simulink model "Task08_Model_Smith"  (R2026a)
settings: Solver=VariableStepAuto
settings Model: Creator=Tommy  LastModifiedBy=Tommy

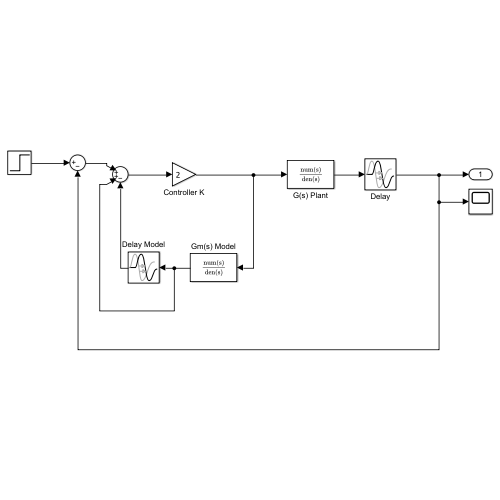
[thumbnail: Simulink's stored preview of the top-level diagram]
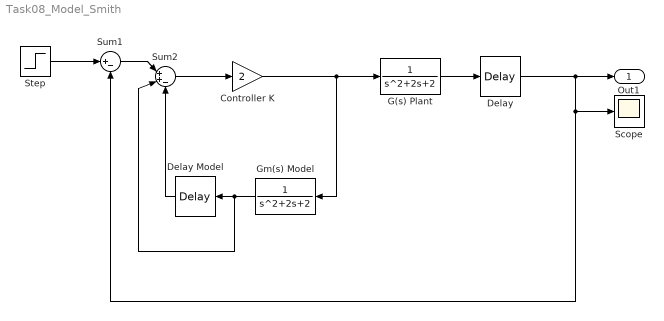
== system Task08_Model_Smith ==
  Controller K : Gain  Gain=2
  Delay : TransportDelay
  Delay Model : TransportDelay
  G(s) Plant : TransferFcn  Denominator=[1 2 2]
  Gm(s) Model : TransferFcn  Denominator=[1 2 2]
  Scope : Scope
  Step : Step  SampleTime=0
  Sum1 : Sum  Inputs=|+-
  Sum2 : Sum  Inputs=|++-
  Out1 : Outport
  wires:
  Sum1/1 -> Sum2/1
  Step/1 -> Sum1/1
  Sum2/1 -> Controller K/1
  Gm(s) Model/1 -> Sum2/2, Delay Model/1
  Controller K/1 -> G(s) Plant/1, Gm(s) Model/1
  Delay/1 -> Out1/1, Sum1/2, Scope/1
  G(s) Plant/1 -> Delay/1
  Delay Model/1 -> Sum2/3
